simulink model "simmodel"  (R2023b)
settings: Solver=VariableStepAuto  StartTime=0.0  StopTime=10.0  RelTol=1e-3
PreLoadFcn:
  | parameters; % Run the script to load parameters into the workspace
StopFcn:
  | %%%plot Euler Angles
  | fig1 = figure();
  | set(fig1,'color','white')
  | p1 = plot(tout,ptpout*180/pi,'-','LineWidth',2);
  | hold on
  | p2 = plot(tout,ptpm*180/pi,'-s','LineWidth',2);
  | p3 = plot(tout,ptpN*180/pi,'--','LineWidth',2);
  | grid on
  | xlabel('Time (sec)')
  | ylabel('Euler Angles (deg)')
  | legend('Phi','Theta','Psi')
  | legend([p1(1),p2(1),p3(1)],'Actual','Measured','Nav')
  | 
  | %%%Plot Angular Velocity
  | fig2 = figure();
  | set(fig2,'color','white')
  | p1=plot(tout,pqrout,'-','LineWidth',2);
  | hold on
  | p2=plot(tout,pqrm,'-s','LineWidth',2);
  | p3=plot(tout,pqrN,'--','LineWidth',2);
  | grid on
  | xlabel('Time (sec)')
  | ylabel('Angular Velocity (rad/s)')
  | legend([p1(1),p2(1),p3(1)],'Actual','Measured','Nav')
  | 
  | %%%Plot the acceleration in reaction wheels
  | fig3 = figure();
  | set(fig3,'color','white')
  | plot(tout,rwa,'LineWidth',2)
  | grid on
  | xlabel('Time (sec)')
  | ylabel('Angular Acceleration RWs (rad/s^2)')
  | legend('X','Y','Z')
  | 
  | %%%Plot the angular velocity of the RWs
  | fig4 = figure();
  | set(fig4,'color','white')
  | plot(tout,w123,'LineWidth',2)
  | grid on
  | xlabel('Time (sec)')
  | ylabel('Angular Velocity of RWs (rad/s)')
  | legend('X','Y','Z')
  | 
  | %%Plot the cube
  | fig = figure();
  | set(fig, 'color', 'white') %white background
  | grid on
  | hold on %new plots added do not delete the existing plot
  | b=l;
  | vertices = [-b/2, -b/2, -b/2;
  |              b/2, -b/2, -b/2;
  |              b/2, b/2, -b/2;
  |              -b/2, b/2, -b/2;
  |              -b/2, -b/2, b/2;
  |              b/2, -b/2, b/2;
  |              b/2, b/2, b/2;
  |              -b/2, b/2, b/2];
  | 
  | faces = [1 2 3 4;
  |          5 6 7 8;
  |          1 2 6 5;
  |          2 3 7 6;
  |          3 4 8 7;
  |          4 1 5 8];
  | 
  | h = patch('Vertices', vertices, 'Faces', faces, 'FaceColor', 'magenta');
  | axis equal;
  | xlabel('X');
  | ylabel('Y');
  | zlabel('Z');
  | view(3);
  | hold on;
  | %
  | % Define reaction wheel diameter and position
  | % wheel_diameter = rr*2; % Half of the length of the cube (cube's length = 2)
  | % theta = linspace(0, 2*pi, 100); % for drawing the circle
  | 
  | % Reaction wheel 1 on the XY plane (Z=b/2)
  | % x1 = wheel_diameter/2 * cos(theta);
  | % y1 = wheel_diameter/2 * sin(theta);
  | % z1 = ones(size(theta)) * b/2; % Top face
  | % rw1 = [x1;y1;z1]';
  | % h1 = plot3(x1, y1, z1, 'r', 'LineWidth', 2);
  | %
  | % % Reaction wheel 2 on the XZ plane (Y=b/2)
  | % y2 = ones(size(theta)) * -b/2; % Side face
  | % z2 = wheel_diameter/2 * cos(theta);
  | % x2 = wheel_diameter/2 * sin(theta);
  | % rw2 = [x2;y2;z2]';
  | % h2 = plot3(x2, y2, z2, 'g', 'LineWidth', 2);
  | %
  | % % Reaction wheel 3 on the YZ plane (X=b/2)
  | % x3 = ones(size(theta)) * -b/2; % Side face
  | % y3 = wheel_diameter/2 * cos(theta);
  | % z3 = wheel_diameter/2 * sin(theta);
  | % rw3 = [x3;y3;z3]';
  | % h3 = plot3(x3, y3, z3, 'b', 'LineWidth', 2);
  | 
  | for i=2:length(ptpout)
  |     Rx = [1 0 0 ; 0 cos(ptpout(i,1)) -sin(ptpout(i,1)) ; 0 sin(ptpout(i,1)) cos(ptpout(i,1))] ;
  |     Ry = [cos(ptpout(i,2)) 0 sin(ptpout(i,2)) ; 0 1 0 ; -sin(ptpout(i,2)) 0 cos(ptpout(i,2))] ;
  |     Rz = [cos(ptpout(i,3)) -sin(ptpout(i,3)) 0 ; sin(ptpout(i,3)) cos(ptpout(i,3)) 0 ; 0 0 1];
  |     coord_new = zeros(8,3);
  |     % rw1_rot = zeros(100,3);
  |     % rw2_rot = zeros(100,3);
  |     % rw3_rot = zeros(100,3);
  |     R = Rz*Ry*Rx;
  |     for j=1:8
  |         coord_new(j,:) = R*vertices(j,:)';
  |     end
  |     % for j=1:100
  |     %     rw1_rot(j,:) = R*rw1(j,:)';
  |     %     rw2_rot(j,:) = R*rw2(j,:)';
  |     %     rw3_rot(j,:) = R*rw3(j,:)';
  |     % end
  |     set(h, 'Vertices', coord_new);
  |     % hold on;
  |     % set(h1, 'XData', rw1_rot(:,1), 'YData', rw1_rot(:,2), 'ZData',rw1_rot(:,3));
  |     % set(h2, 'XData', rw2_rot(:,1), 'YData', rw2_rot(:,2), 'ZData',rw2_rot(:,3));
  |     % set(h3, 'XData', rw3_rot(:,1), 'YData', rw3_rot(:,2), 'ZData',rw3_rot(:,3));
  |     %hold off
  |     drawnow;
  |     vertices = coord_new;
  |     % rw1 = rw1_rot;
  |     % rw2 = rw2_rot;
  |     % rw3 = rw3_rot;
  |     pause(0.5);
  | 
  | end
values from neighbouring files (symbols this model uses):
  g = 9.81    [Cube.m]    (also in parameters.m)
  gamma = [1 1 -1 0; 1 -1 0 1; -1 0 -1 1; 0 1 1 1]    [Cube.m]    (also in parameters.m)
  Ic_bar = (IcO - Iw)    [parameters.m]    (also in paramters.m = IcO - Iw)
  invIc_bar = inv(Ic_bar)    [parameters.m]
  invIw = inv(Iw)    [parameters.m]
  Iw = [Iwxx 0 0; 0 Iwxx 0; 0 0 Iwxx]    [parameters.m]    (also in paramters.m; reaction_wheel_params.m)
  l = 0.15    [parameters.m]    (also in paramters.m)
  mc_bar = ms + 2*mw    [Cube.m]    (also in parameters.m = 0.74)
  pqrm = zeros(length(tout),3)    [main.m]
  pqrN = zeros(length(tout),3)    [main.m]
  pqrout = stateout(:,11:13)    [main.m]
  ptpout = Quaternions2EulerAngles(q0123out)    [main.m]
  tout = 0:timestep:tfinal    [main.m]
libraries: aerolibutil x7, matrix_library x3, sharedutil x1, vrlib x1
settings Model: Creator=kriti  LastModifiedBy=kriti

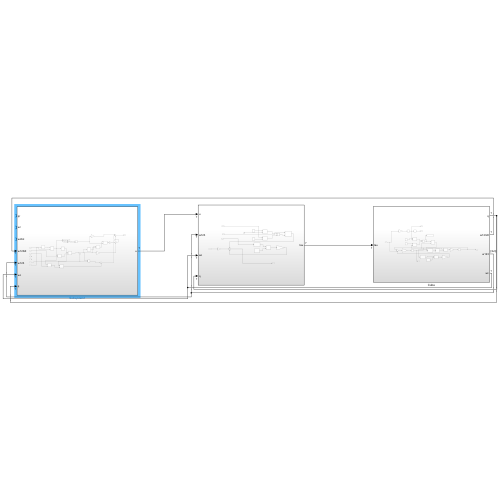
[thumbnail: Simulink's stored preview of the top-level diagram]
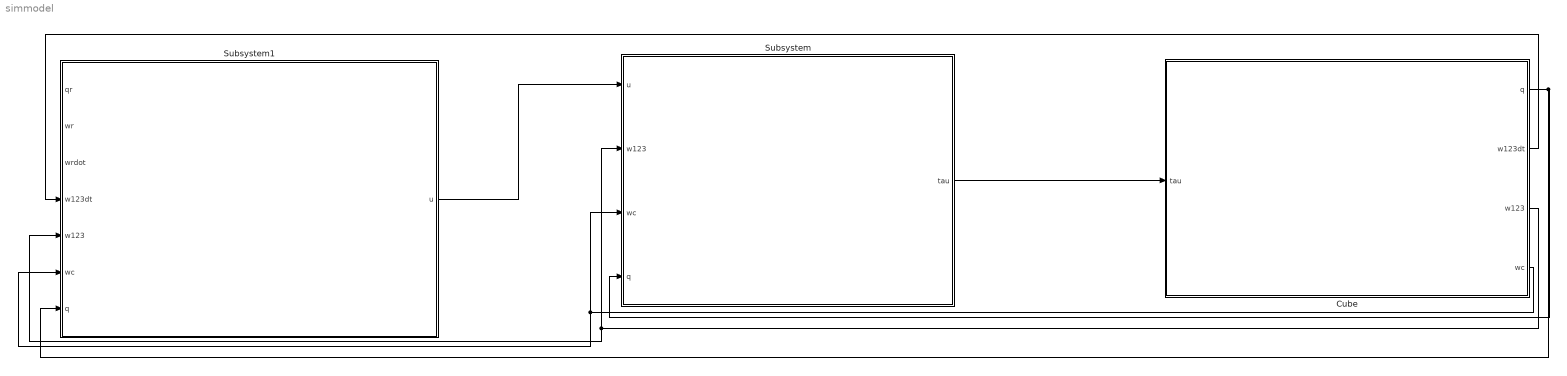
== system simmodel ==
  Cube : Subsystem
  Subsystem : Subsystem
  Subsystem1 : Subsystem
  wires:
  Cube/1(q) -> Subsystem1/7(q), Subsystem/4(q)
  Cube/3(w123) -> Subsystem/2(w123), Subsystem1/5(w123)
  Cube/4(wc) -> Subsystem/3(wc), Subsystem1/6(wc)
  Subsystem/1(tau) -> Cube/1(tau)
  Subsystem1/1(u) -> Subsystem/1(u)
  Cube/2(w123dt) -> Subsystem1/4(w123dt)

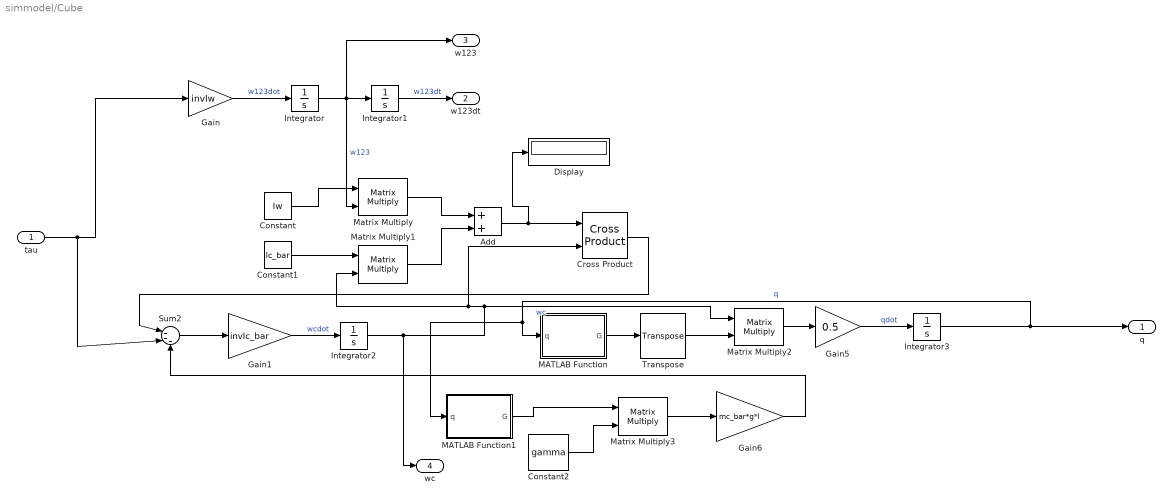
== system simmodel/Cube ==
  tau : Inport
  Add : Sum
  Constant : Constant  Value=Iw
  Constant1 : Constant  Value=Ic_bar
  Constant2 : Constant  Value=gamma
  Cross Product : matrix_library/Cross Product
  Display : Display
  Gain : Gain  Gain=invIw
  Gain1 : Gain  Gain=invIc_bar
  Gain5 : Gain  Gain=0.5
  Gain6 : Gain  Gain=mc_bar*g*l
  Integrator{,1..3} (4 alike) : Integrator
  MATLAB Function : MATLAB Function  TreatAsAtomicUnit=on
  MATLAB Function1 : MATLAB Function  TreatAsAtomicUnit=on
  Matrix Multiply{,1..3} (4 alike) : Product  Multiplication=Matrix(*)
  Sum2 : Sum  Inputs=|---
  Transpose : matrix_library/Transpose
  q : Outport
  w123dt : Outport  Port=2
  w123 : Outport  Port=3
  wc : Outport  Port=4
  wires:
  Gain/1 -> Integrator/1  "w123dot"
  Integrator/1 -> Matrix Multiply/2, w123/1, Integrator1/1  "w123"
  Integrator1/1 -> w123dt/1  "w123dt"
  Constant/1 -> Matrix Multiply/1
  Sum2/1 -> Gain1/1
  Gain1/1 -> Integrator2/1  "wcdot"
  Integrator2/1 -> wc/1, Cross Product/2, Matrix Multiply1/2, Matrix Multiply2/1  "wc"
  Constant1/1 -> Matrix Multiply1/1
  Matrix Multiply/1 -> Add/1
  Matrix Multiply1/1 -> Add/2
  Add/1 -> Display/1, Cross Product/1
  Cross Product/1 -> Sum2/1
  MATLAB Function/1(G) -> Transpose/1
  Transpose/1 -> Matrix Multiply2/2
  Matrix Multiply2/1 -> Gain5/1
  Gain5/1 -> Integrator3/1  "qdot"
  Integrator3/1 -> MATLAB Function1/1(q), MATLAB Function/1(q), q/1  "q"
  MATLAB Function1/1(G) -> Matrix Multiply3/1
  Constant2/1 -> Matrix Multiply3/2
  Matrix Multiply3/1 -> Gain6/1
  Gain6/1 -> Sum2/3
  tau/1 -> Sum2/2, Gain/1

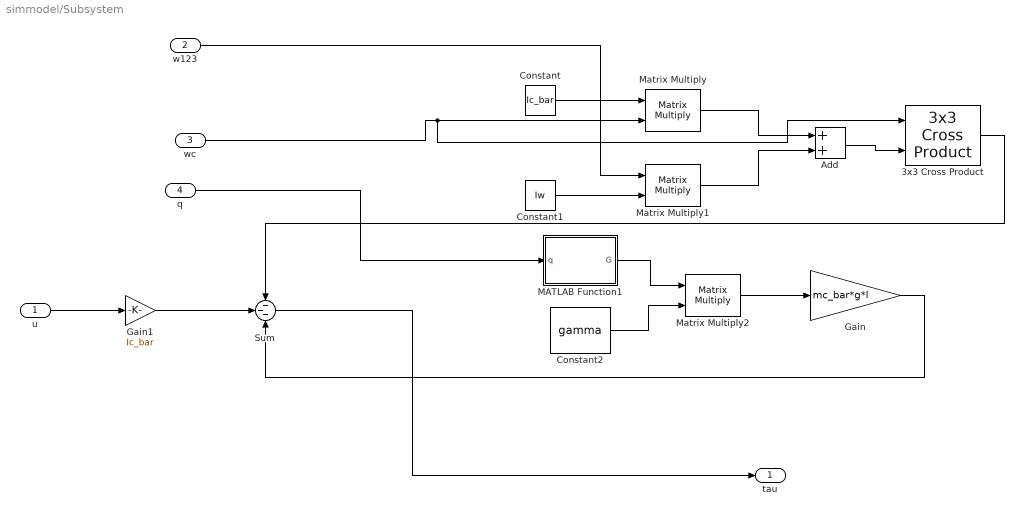
== system simmodel/Subsystem ==
  u : Inport
  w123 : Inport  Port=2
  wc : Inport  Port=3
  q : Inport  Port=4
  3x3 Cross Product : sharedutil/3x3 Cross Product  aMode=aMode
      settings: LibrarySourceBlock=aerolibutil/3x3 Cross Product
  Add : Sum
  Constant : Constant  Value=Ic_bar  VectorParams1D=off
  Constant1 : Constant  Value=Iw
  Constant2 : Constant  Value=gamma
  Gain : Gain  Gain=mc_bar*g*l
  Gain1 : Gain  Gain=Ic_bar
  MATLAB Function1 : MATLAB Function  TreatAsAtomicUnit=on
  Matrix Multiply : Product  Multiplication=Matrix(*)
  Matrix Multiply1 : Product  Multiplication=Matrix(*)
  Matrix Multiply2 : Product  Multiplication=Matrix(*)
  Sum : Sum  Inputs=---
  tau : Outport
  wires:
  Constant/1 -> Matrix Multiply/1
  wc/1 -> 3x3 Cross Product/1, Matrix Multiply/2
  Constant1/1 -> Matrix Multiply1/2
  w123/1 -> Matrix Multiply1/1
  Matrix Multiply/1 -> Add/1
  Matrix Multiply1/1 -> Add/2
  Add/1 -> 3x3 Cross Product/2
  MATLAB Function1/1(G) -> Matrix Multiply2/1
  q/1 -> MATLAB Function1/1(q)
  Constant2/1 -> Matrix Multiply2/2
  Matrix Multiply2/1 -> Gain/1
  3x3 Cross Product/1 -> Sum/1
  Gain/1 -> Sum/3
  Sum/1 -> tau/1
  u/1 -> Gain1/1
  Gain1/1 -> Sum/2

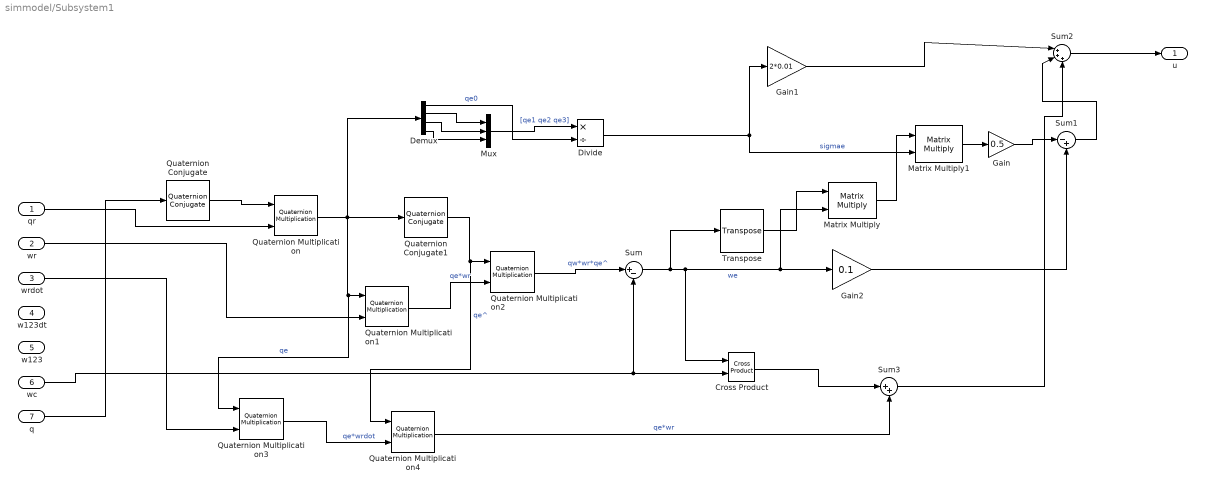
== system simmodel/Subsystem1 ==
  qr : Inport
  wr : Inport  Port=2
  wrdot : Inport  Port=3
  w123dt : Inport  Port=4
  w123 : Inport  Port=5
  wc : Inport  Port=6
  q : Inport  Port=7
  Cross Product : vrlib/Utilities/Cross Product
  Demux : Demux
  Divide : Product  Inputs=*/
  Gain : Gain  Gain=0.5
  Gain1 : Gain  Gain=2*0.01
  Gain2 : Gain  Gain=0.1
  Matrix Multiply : Product  Multiplication=Matrix(*)
  Matrix Multiply1 : Product  Multiplication=Matrix(*)
  Mux : Mux  Inputs=3
  Quaternion Conjugate : aerolibutil/Quaternion Conjugate
  Quaternion Conjugate1 : aerolibutil/Quaternion Conjugate
  Quaternion Multiplication{,1..4} (5 alike) : aerolibutil/Quaternion Multiplication
  Sum : Sum  Inputs=|+-
  Sum1 : Sum  Inputs=|-+
  Sum2 : Sum  Inputs=|+++
  Sum3 : Sum  Inputs=|++
  Transpose : matrix_library/Transpose
  u : Outport
  wires:
  q/1 -> Quaternion Conjugate/1
  Quaternion Conjugate/1 -> Quaternion Multiplication/1
  qr/1 -> Quaternion Multiplication/2
  Quaternion Multiplication/1 -> Demux/1, Quaternion Conjugate1/1, Quaternion Multiplication3/1, Quaternion Multiplication1/1  "qe"
  wr/1 -> Quaternion Multiplication1/2
  Quaternion Conjugate1/1 -> Quaternion Multiplication4/1, Quaternion Multiplication2/1  "qe^"
  Quaternion Multiplication1/1 -> Quaternion Multiplication2/2  "qe*wr"
  wrdot/1 -> Quaternion Multiplication3/2
  Quaternion Multiplication3/1 -> Quaternion Multiplication4/2  "qe*wrdot"
  wc/1 -> Sum/2, Cross Product/2
  Quaternion Multiplication2/1 -> Sum/1  "qw*wr*qe^"
  Sum/1 -> Transpose/1, Gain2/1, Matrix Multiply/2, Cross Product/1  "we"
  Demux/2 -> Mux/1
  Demux/3 -> Mux/2
  Demux/4 -> Mux/3
  Mux/1 -> Divide/1  "[qe1 qe2 qe3]"
  Demux/1 -> Divide/2  "qe0"
  Divide/1 -> Gain1/1, Matrix Multiply1/2  "sigmae"
  Transpose/1 -> Matrix Multiply/1
  Matrix Multiply/1 -> Matrix Multiply1/1
  Matrix Multiply1/1 -> Gain/1
  Gain/1 -> Sum1/1
  Gain2/1 -> Sum1/2
  Gain1/1 -> Sum2/1
  Sum1/1 -> Sum2/2
  Cross Product/1 -> Sum3/1
  Quaternion Multiplication4/1 -> Sum3/2  "qe*wr"
  Sum3/1 -> Sum2/3
  Sum2/1 -> u/1

== matlab function simmodel/Cube/MATLAB Function ==
  data: q input; G output
function G = computeG(q)
    q0 = q(1); q1 = q(2); q2 = q(3); q3 = q(4);
    q_vector = [q1; q2; q3];
    q_skew = [0 -q3 q2; q3 0 -q1; q2 q1 0];
    G = [q_vector q0*eye(3) - q_skew];
end

== matlab function simmodel/Subsystem/MATLAB Function1 ==
  data: q input; G output
function G = computeG(q)
    q0 = q(1); q1 = q(2); q2 = q(3); q3 = q(4);
    q_vector = [q1; q2; q3];
    q_skew = [0 -q3 q2; q3 0 -q1; q2 q1 0];
    G = [q_vector q0*eye(3) - q_skew];
end

== matlab function simmodel/Cube/MATLAB Function1 ==
  data: q input; G output
function G = computeG(q)
    q0 = q(1); q1 = q(2); q2 = q(3); q3 = q(4);
    q_vector = [q1; q2; q3];
    q_skew = [0 -q3 q2; q3 0 -q1; q2 q1 0];
    G = [q_vector q0*eye(3) - q_skew];
end
